simulink model "Modelo_Parcial_S5_2019b"  (R2019b)
settings: Solver=VariableStepAuto  StartTime=0.0  StopTime=0.05  RelTol=1e-3
undefined symbols (not defined in the file or in its folder): A, B_mat, C, D
settings DebuggingCC: UnconnectedInputMsg=none  UnconnectedOutputMsg=none  UnconnectedLineMsg=none
settings ModelReferenceCC: UpdateModelReferenceTargets=IfOutOfDate  EnableRefExpFcnMdlSchedulingChecks=off
settings RTWCC: Description=Generic Real-Time Target
settings ConfigComp: CovBoundaryAbsTol=1.0e-5

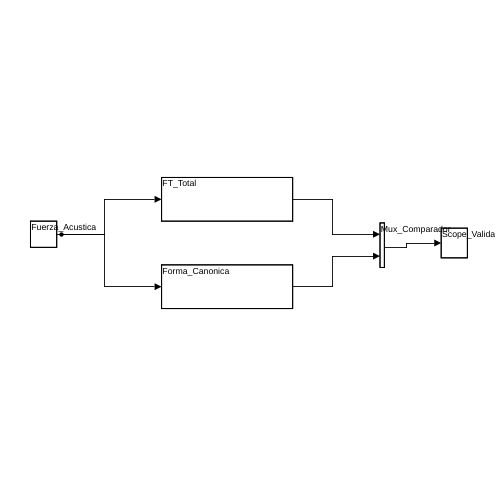
[thumbnail: Simulink's stored preview of the top-level diagram]
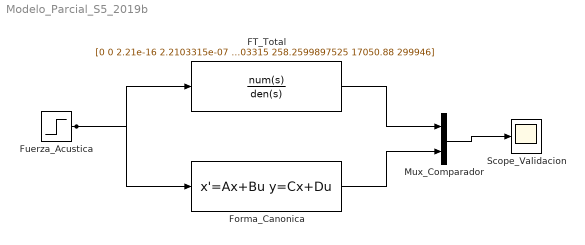
== system Modelo_Parcial_S5_2019b ==
  FT_Total : TransferFcn  Numerator=[0 0 2.21e-16 2.2103315e-07 0.033250001105 16.105 500]  Denominator=[2.21e-20 2.210663e-11 6.640497471e-06 0.50047103315 258.2599897525 17050.88 299946]
  Forma_Canonica : StateSpace  A=A  B=B_mat  C=C  D=D  InitialCondition=0
  Fuerza_Acustica : Step  Time=0  After=0.001  SampleTime=0
  Mux_Comparador : Mux  Inputs=2
  Scope_Validacion : Scope
  wires:
  Fuerza_Acustica/1 -> FT_Total/1, Forma_Canonica/1
  FT_Total/1 -> Mux_Comparador/1
  Forma_Canonica/1 -> Mux_Comparador/2
  Mux_Comparador/1 -> Scope_Validacion/1
